simulink model "ssm_airframe"  (R2022a)
settings: Solver=ode45  StartTime=0.0  StopTime=SimTime  RelTol=1e-3  AbsTol=1e-6
PreLoadFcn:
  | airframe_init
StopFcn:
  | % airframe_plot
values from neighbouring files (symbols this model uses):
  boosting_time = 5    [airframe_init.m]
  thrust_magnitude = 78*1e+3    (= 78000)    [airframe_init.m]
libraries: shared6dof x1, simulink x1
settings Model: Creator=amani  LastModifiedBy=amani

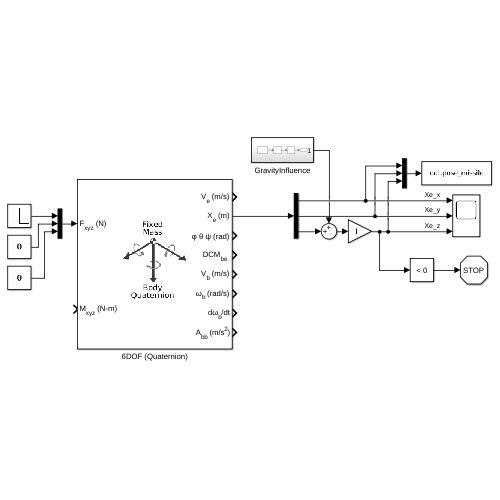
[thumbnail: Simulink's stored preview of the top-level diagram]
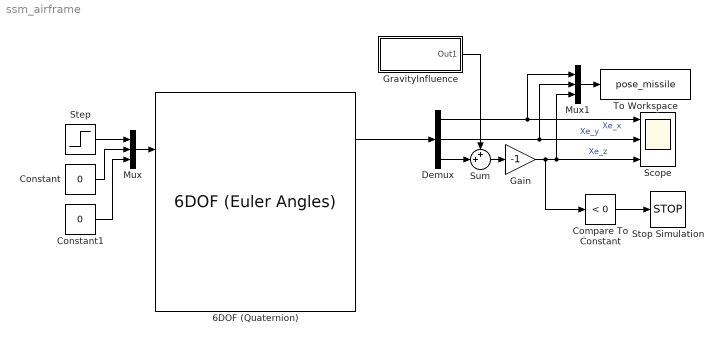
== system ssm_airframe ==
  6DOF (Quaternion) : shared6dof/6DOF (Euler Angles)  units=Metric (MKS)  mtype=Fixed  rep=Quaternion  xme_0=pose_ini  Vm_0=vel_ini  eul_0=rot_ini  pm_0=rotvel_ini  mass_0=mass  mass_e=0.5  mass_f=2.0  inertia=inertia  inertia_e=eye(3)  inertia_f=2*eye(3)  k_quat=1.0  vre_flag=on  abi_flag=off  aMode=0  xme_statename=''  Vm_statename=''  eul_statename=''  quat_statename=''  pm_statename=''  mass_statename=''
      settings: SourceProductBaseCode=AE,PW,DR,MT,VE
  Compare To Constant : simulink/Logic and Bit Operations/Compare To Constant  relop=<  const=0  OutDataTypeStr=boolean
  Constant : Constant  Value=0
  Constant1 : Constant  Value=0
  Demux : Demux  Outputs=3
  Gain : Gain  Gain=-1
  GravityInfluence : Subsystem
  Mux : Mux  Inputs=3
  Mux1 : Mux  Inputs=3
  Scope : Scope  NumInputPorts=3
  Step : Step  Time=boosting_time  Before=thrust_magnitude  After=0  SampleTime=0
  Stop Simulation : Stop
  Sum : Sum  Inputs=++|
  To Workspace : ToWorkspace  VariableName=pose_missile  SaveFormat=Structure With Time  SampleTime=-1
  wires:
  Constant/1 -> Mux/2
  Mux/1 -> 6DOF (Quaternion)/1
  6DOF (Quaternion)/2 -> Demux/1
  Gain/1 -> Scope/3, Mux1/3, Compare To Constant/1  "Xe_z"
  Sum/1 -> Gain/1
  Compare To Constant/1 -> Stop Simulation/1
  Demux/2 -> Scope/2, Mux1/2  "Xe_y"
  Demux/1 -> Scope/1, Mux1/1  "Xe_x"
  Constant1/1 -> Mux/3
  Step/1 -> Mux/1
  Mux1/1 -> To Workspace/1
  GravityInfluence/1(Out1) -> Sum/1
  Demux/3 -> Sum/2

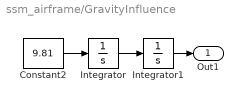
== system ssm_airframe/GravityInfluence ==
  Constant2 : Constant  Value=9.81
  Integrator : Integrator
  Integrator1 : Integrator
  Out1 : Outport
  wires:
  Integrator/1 -> Integrator1/1
  Constant2/1 -> Integrator/1
  Integrator1/1 -> Out1/1
